simulink library "tco"  (Simulink 8.1)
settings: Solver=ode1  StartTime=0.0  StopTime=Inf  FixedStep=0.001  RelTol=1e-3
PostLoadFcn:
  | , if any(exist('dsrtsu_mdlpostloadfcn', 'file') == [2, 3, 6]), try dsrtsu_mdlpostloadfcn('Execute', bdroot); catch fprintf('Error in PostLoadFcn (dsrtsu_mdlpostloadfcn) for model "%s":\n %s\n', bdroot, lasterr); end, end,
libraries: dit x1, tgt x1
settings Model: DSRTSU_INTERNAL_RTI_VER=450  DSRTSU_INTERNAL_RTI_TYPE=rti1401  RTICANMMDATA=struct('GeneralSetupData',struct('modelroot','D:\ELN150201_TAIWAN\trunk\AdasDragon\software\sw_development\arch\app\acc','generalsettings',struct('filesettings',struct('destfolder',struct('Name','RTICANMM_FILES','Check',1),'buildfolder',struct('Name','.','Check',1),'AbsDestfolder',struct('Name','D:\ELN150201_TAIWAN\trunk\AdasDragon\software\sw_development\arch\app\acc\RTICANMM_FILES'),'AbsBuildfolder',struct('Name','D:\ELN150201_TAIWAN\trunk\AdasDragon\software\sw_development\arch\app\acc'))),'options',struct('addpaths',1,'rmpaths',1,'addtrcexclusion',logical(1),'cannavigator',struct('checkmonitoring',0),'show_usrtrc',0,'use_usrtrc',0),'advanced',struct('options',[1 1 1 1 1 1 1 1 1 1 1 1 1 1 1 1 1 1 1 1 1 1 1 1 1 1 1 1 1 1 1 1 1 1 1 1 1 1 1 1 1 1 1 1 1 1 1 1 1 1 1 1 1 1 1 1 1 1 1 1 1 1 1 1 1 1 1 1 1 1 1 1 1 1 1 1 1 1 1 1 1 1 1 1 1 1 1 1 1 1 1 1 1 1 1 1 1 1 1 1]),'MPSetup',{{}},'modelname','tco','block','tco'))  DSRTSU_INTERNAL_RTIFPGA=40  Creator=AT015411  LastModifiedBy=AT015555

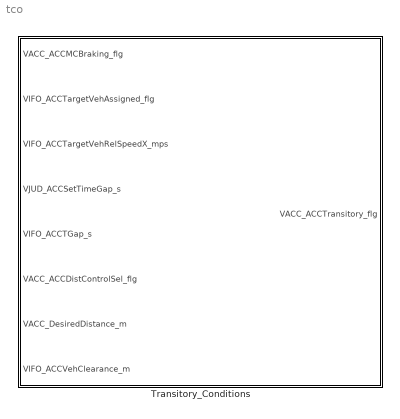
== system tco ==
  Transitory_Conditions : Subsystem

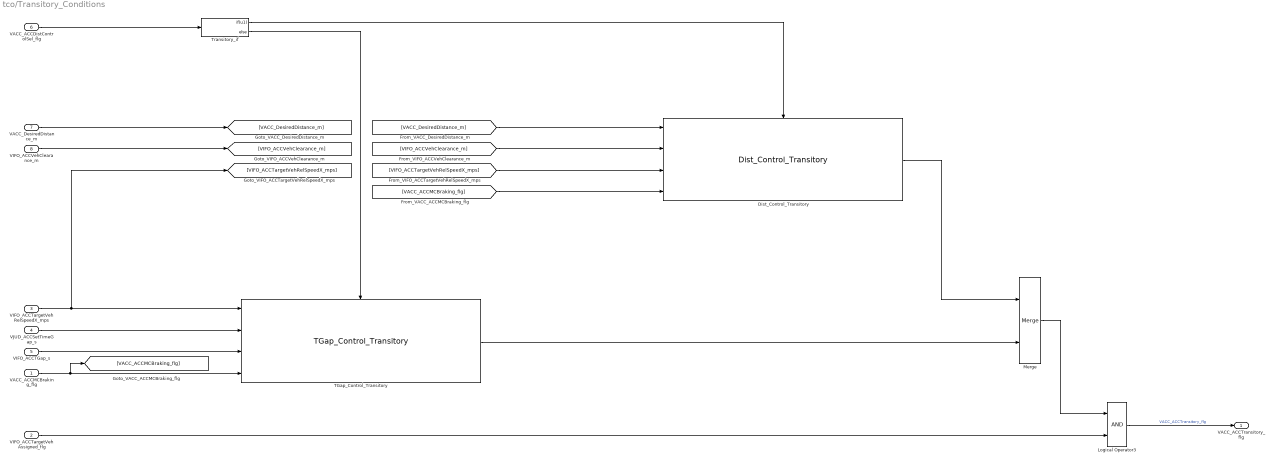
== system tco/Transitory_Conditions ==
  VACC_ACCMCBraking_flg : Inport
  VIFO_ACCTargetVehAssigned_flg : Inport  Port=2
  VIFO_ACCTargetVehRelSpeedX_mps : Inport  Port=3
  VJUD_ACCSetTimeGap_s : Inport  Port=4
  VIFO_ACCTGap_s : Inport  Port=5
  VACC_ACCDistControlSel_flg : Inport  Port=6
  VACC_DesiredDistance_m : Inport  Port=7
  VIFO_ACCVehClearance_m : Inport  Port=8
  Dist_Control_Transitory : dit/Dist_Control_Transitory
  Logical Operator3 : Logic  AllPortsSameDT=off  OutDataTypeStr=boolean
  Merge : Merge
  TGap_Control_Transitory : tgt/TGap_Control_Transitory
  Transitory_if : If  IfExpression=u1
  VACC_ACCTransitory_flg : Outport
  wires:
  Merge/1 -> Logical Operator3/1
  TGap_Control_Transitory/1 -> Merge/2
  Dist_Control_Transitory/1 -> Merge/1
  Transitory_if/2 -> TGap_Control_Transitory/Action
  Transitory_if/1 -> Dist_Control_Transitory/Action
  VIFO_ACCVehClearance_m/1 -> [VIFO_ACCVehClearance_m]
  VACC_DesiredDistance_m/1 -> [VACC_DesiredDistance_m]
  VACC_ACCMCBraking_flg/1 -> TGap_Control_Transitory/4, [VACC_ACCMCBraking_flg]
  VIFO_ACCTargetVehRelSpeedX_mps/1 -> [VIFO_ACCTargetVehRelSpeedX_mps], TGap_Control_Transitory/1
  VACC_ACCDistControlSel_flg/1 -> Transitory_if/1
  Logical Operator3/1 -> VACC_ACCTransitory_flg/1  "VACC_ACCTransitory_flg"
  VIFO_ACCTargetVehAssigned_flg/1 -> Logical Operator3/2
  VJUD_ACCSetTimeGap_s/1 -> TGap_Control_Transitory/2
  VIFO_ACCTGap_s/1 -> TGap_Control_Transitory/3
  [VACC_ACCMCBraking_flg] -> Dist_Control_Transitory/4
  [VIFO_ACCTargetVehRelSpeedX_mps] -> Dist_Control_Transitory/3
  [VIFO_ACCVehClearance_m] -> Dist_Control_Transitory/2
  [VACC_DesiredDistance_m] -> Dist_Control_Transitory/1
